simulink model "testing"  (R2024b)
settings: Solver=FixedStepAuto  StartTime=0.0  StopTime=100  FixedStep=1/10  RelTol=1e-3
libraries: hdlsllib x2
settings Model: Creator=UTSAB KARAN  LastModifiedBy=UTSAB KARAN

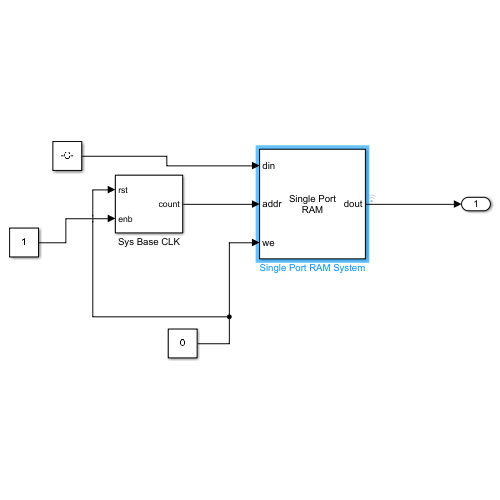
[thumbnail: Simulink's stored preview of the top-level diagram]
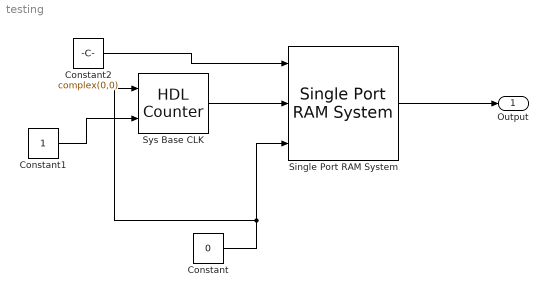
== system testing ==
  Constant : Constant  Value=0  OutDataTypeStr=boolean
  Constant1 : Constant  OutDataTypeStr=boolean
  Constant2 : Constant  Value=complex(0,0)  OutDataTypeStr=fixdt(1,8,6)
  Single Port RAM System : hdlsllib/HDL RAMs/Single Port RAM System  RAMType=Single port  AsyncRead=off  WriteOutputValue=New data  RAMInitialValue=ram1_init_data  allowBusInputs=off  WritesHaveOutput=on  NumReads=0  NumWrites=1  SimulateUsing=Code generation  ModelRAMDelay=on
  Sys Base CLK : hdlsllib/Sources/HDL Counter  CountType=Count limited  CountInit=0  CountStep=1  CountMax=1000  CountFromType=Initial value  CountFrom=0  CountResetPort=on  CountLoadPort=off  CountEnbPort=on  CountDirPort=off  CountHitOutputPort=off  CountDataType=Unsigned  CountWordLen=12  CountFracLen=0  CountSampTime=1
  Output : Outport  OutDataTypeStr=fixdt(1,8,6)
  wires:
  Constant/1 -> Sys Base CLK/1, Single Port RAM System/3
  Single Port RAM System/1 -> Output/1
  Sys Base CLK/1 -> Single Port RAM System/2
  Constant1/1 -> Sys Base CLK/2
  Constant2/1 -> Single Port RAM System/1
